simulink model "MoboticStartup_TimingSync"  (R2024a)
settings: Solver=FixedStepAuto  StartTime=0.0  StopTime=inf  FixedStep=tstep  RelTol=1e-3
settings Model: DataDictionary=configuration_dictionary.sldd  Creator=matlab.cut  LastModifiedBy=matlab.cut
settings SolverCC: ConcurrentTasks=on  PositivePriorityOrder=on
settings OptimizationCC: BlockReduction=off  DefaultParameterBehavior=Inlined  OptimizeBlockIOStorage=off
settings DebuggingCC: TasksWithSamePriorityMsg=none
settings HardwareCC: ProdBitPerLong=64  ProdLongLongMode=on  ProdHWDeviceType=Intel->x86-64 (Linux 64)
settings ModelReferenceCC: ModelReferenceNumInstancesAllowed=Single
settings SFSimCC: MATLABDynamicMemAlloc=off
settings RTWCC: Description=Speedgoat Real-Time Target Machine  SystemTargetFile=speedgoat.tlc  TemplateMakefile=slrealtime_default_tmf  Toolchain=Simulink Real-Time Toolchain  BuildConfiguration=Faster Runs  CodeExecutionProfiling=on  TargetLang=C++
settings CodeAppCC: MaxIdLength=127
settings SimulinkRealTimeTargetCC: InstructionSetFMA=off  LogToMDFFile=off

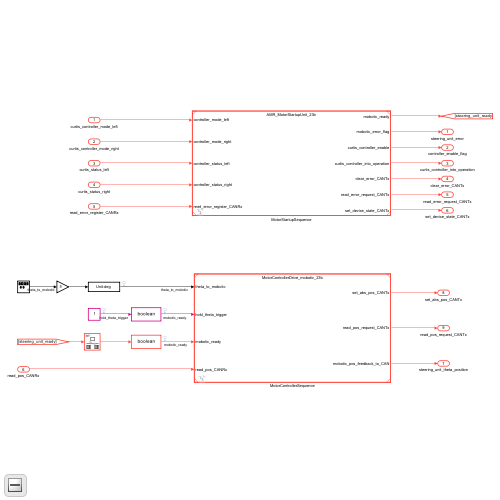
[thumbnail: Simulink's stored preview of the top-level diagram]
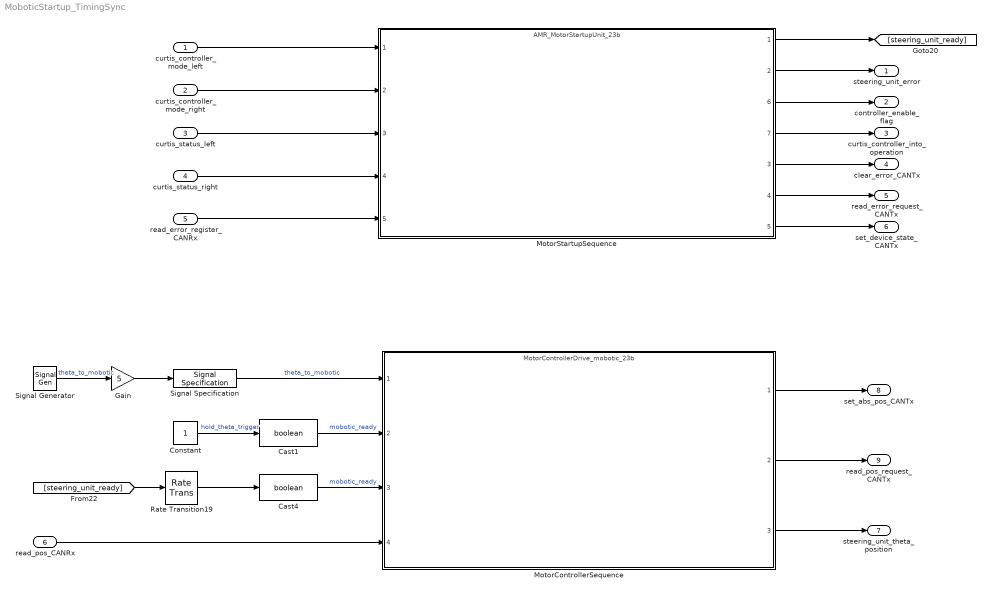
== system MoboticStartup_TimingSync ==
  curtis_controller_mode_left : Inport
  curtis_controller_mode_right : Inport  Port=2
  curtis_status_left : Inport  Port=3
  curtis_status_right : Inport  Port=4
  read_error_register_CANRx : Inport  Port=5
  read_pos_CANRx : Inport  Port=6
  Cast1 : DataTypeConversion  OutDataTypeStr=boolean  SaturateOnIntegerOverflow=off  RndMeth=Floor
  Cast4 : DataTypeConversion  OutDataTypeStr=boolean  SaturateOnIntegerOverflow=off  RndMeth=Floor
  Constant : Constant
  Gain : Gain  Gain=5
  MotorControllerSequence : ModelReference  ModelNameDialog=MotorControllerDrive_mobotic_23b.slx  SimulationMode=Normal  ModelReferenceVersion=2.16
  MotorStartupSequence : ModelReference  ModelNameDialog=AMR_MotorStartupUnit_23b.slx  SimulationMode=Normal  ModelReferenceVersion=2.18
      settings: PortSchema="{\"entries\":[{\"content\":{\"sides\":[{\"content\":{\"connectorIds\":[\"In1\",\"In2\",\"In3\",\"In4\",\"In5\"]},\"type\":\"ConnectorPlacement.EquallySpacedRectSide\",\"uuid\":\"3921406d-efe8-4d43-b839-8e6950b3e7d6\"},{\"content\":{\"connectorIds\":[\"Out1\",\"Out2\",\"Out6\",\"Out7\",\"Out3\",\"Out4\",\"Out5\"],\"side\":\"RIGHT\"},\"type\":\"ConnectorPlacement.EquallySpacedRectSide\",\"uuid\":\"6c47fb42-e1f1-4a89-878d-326b7208c2c9\"},{\"content\":{\"side\":\"TOP\"},\"type\":\"ConnectorPlacement.EquallySpacedRectSide\",\"uuid\":\"d0ee5206-f0b1-4520-be60-f9f02d74dabf\"}]},\"type\":\"ConnectorPlacement.EquallySpacedConnector\",\"uuid\":\"950d4306-13c4-4234-b648-b593fc60393c\"}],\"packageUris\":[\"http://schema.mathworks.com/mf0/Connector/R2020b\"],\"version\":\"1.0\"}"
  Rate Transition19 : RateTransition
  Signal Generator : SignalGenerator  Frequency=0.1
  Signal Specification : SignalSpecification  Unit=deg
  steering_unit_error : Outport
  controller_enable_flag : Outport  Port=2
  curtis_controller_into_operation : Outport  Port=3
  clear_error_CANTx : Outport  Port=4
  read_error_request_CANTx : Outport  Port=5
  set_device_state_CANTx : Outport  Port=6
  steering_unit_theta_position : Outport  Port=7
  set_abs_pos_CANTx : Outport  Port=8
  read_pos_request_CANTx : Outport  Port=9
  wires:
  MotorStartupSequence/4 -> read_error_request_CANTx/1
  MotorStartupSequence/6 -> controller_enable_flag/1
  MotorStartupSequence/5 -> set_device_state_CANTx/1
  MotorStartupSequence/3 -> clear_error_CANTx/1
  curtis_controller_mode_left/1 -> MotorStartupSequence/1
  curtis_controller_mode_right/1 -> MotorStartupSequence/2
  MotorStartupSequence/2 -> steering_unit_error/1
  read_error_register_CANRx/1 -> MotorStartupSequence/5
  MotorStartupSequence/7 -> curtis_controller_into_operation/1
  curtis_status_right/1 -> MotorStartupSequence/4
  curtis_status_left/1 -> MotorStartupSequence/3
  MotorStartupSequence/1 -> [steering_unit_ready]
  Constant/1 -> Cast1/1  "hold_theta_trigger"
  read_pos_CANRx/1 -> MotorControllerSequence/4
  Rate Transition19/1 -> Cast4/1
  Cast4/1 -> MotorControllerSequence/3  "mobotic_ready"
  [steering_unit_ready] -> Rate Transition19/1
  Signal Generator/1 -> Gain/1  "theta_to_mobotic"
  Signal Specification/1 -> MotorControllerSequence/1  "theta_to_mobotic"
  Gain/1 -> Signal Specification/1
  Cast1/1 -> MotorControllerSequence/2  "mobotic_ready"
  MotorControllerSequence/3 -> steering_unit_theta_position/1
  MotorControllerSequence/2 -> read_pos_request_CANTx/1
  MotorControllerSequence/1 -> set_abs_pos_CANTx/1
